simulink model "model_InputConditioningAutoStop"  (R2024a)
settings: Solver=FixedStepAuto  StartTime=0.0  StopTime=10.0  RelTol=1e-3
settings Model: Creator=Gabriel  LastModifiedBy=Gabriel

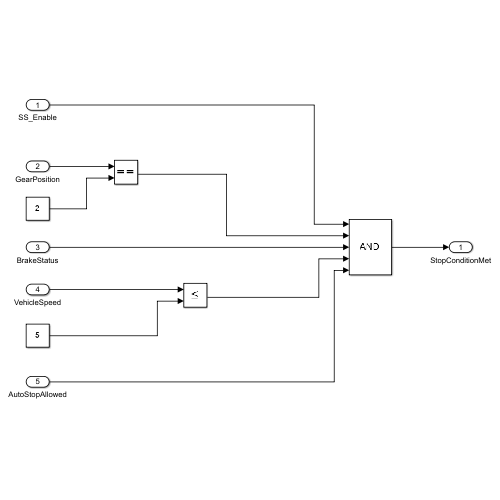
[thumbnail: Simulink's stored preview of the top-level diagram]
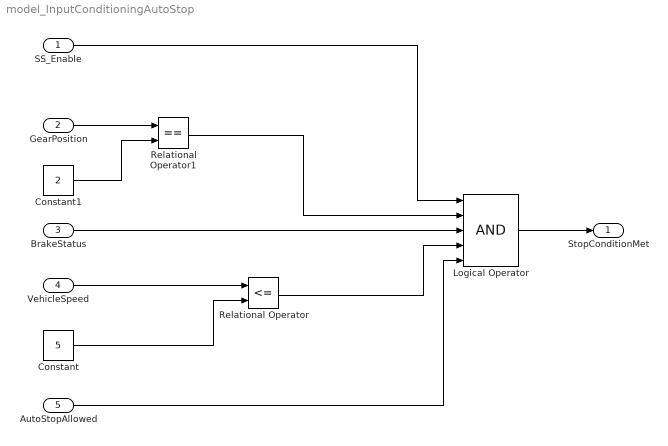
== system model_InputConditioningAutoStop ==
  SS_Enable : Inport
  GearPosition : Inport  Port=2
  BrakeStatus : Inport  Port=3
  VehicleSpeed : Inport  Port=4
  AutoStopAllowed : Inport  Port=5
  Constant : Constant  Value=5
  Constant1 : Constant  Value=2
  Logical Operator : Logic  Inputs=5  AllPortsSameDT=off  OutDataTypeStr=boolean
  Relational Operator : RelationalOperator  Operator=<=  OutDataTypeStr=boolean  RndMeth=Simplest  InputSameDT=off
  Relational Operator1 : RelationalOperator  Operator===  OutDataTypeStr=boolean  RndMeth=Simplest  InputSameDT=off
  StopConditionMet : Outport
  wires:
  Constant1/1 -> Relational Operator1/2
  AutoStopAllowed/1 -> Logical Operator/5
  Relational Operator1/1 -> Logical Operator/2
  Relational Operator/1 -> Logical Operator/4
  GearPosition/1 -> Relational Operator1/1
  SS_Enable/1 -> Logical Operator/1
  BrakeStatus/1 -> Logical Operator/3
  VehicleSpeed/1 -> Relational Operator/1
  Constant/1 -> Relational Operator/2
  Logical Operator/1 -> StopConditionMet/1
